simulink model "rpend_devdriv"  (R2018b)
settings: Solver=FixedStepDiscrete  StartTime=0.0  StopTime=999  FixedStep=0.01  RelTol=1e-3  EnableMultiTasking=on
values from neighbouring files (symbols this model uses):
  J = 0.000115    [init2.m]    (also in run_simulink_model.m)
  K = lqr(A, B, Q, R)    [run_simulink_model.m]
  mgl = 4    [init2.m]    (also in run_simulink_model.m)
  SP = [0,0,0,0]    [init2.m]    (also in run_simulink_model.m = [0, 0, 0, 0])
settings Model: SimulationMode=external  ExtModeTrigDuration=30000  Creator=user  LastModifiedBy=Student
settings DataIOCC: SaveFormat=Array  SignalLoggingSaveFormat=ModelDataLogs
settings OptimizationCC: ExpressionDepthLimit=2147483647  LifeSpan=inf
settings DebuggingCC: UnderspecifiedInitializationDetection=Classic  MergeDetectMultiDrivingBlocksExec=none  SolverPrmCheckMsg=warning  FcnCallInpInsideContextMsg=warning  StateNameClashWarn=warning  SFUnexpectedBacktrackingDiag=warning  SFNoUnconditionalDefaultTransitionDiag=warning  SFExecutionAtInitializationDiag=none
settings HardwareCC: ProdBitPerPointer=32  ProdBitPerSizeT=32  ProdBitPerPtrDiffT=32  ProdLargestAtomicFloat=None  ProdIntDivRoundTo=Undefined  ProdEndianess=Unspecified  ProdWordSize=32  ProdHWDeviceType=32-bit Generic
settings ModelReferenceCC: PropagateSignalLabelsOutOfModel=off
settings SFSimCC: SimUseLocalCustomCode=off
settings RTWCC: SystemTargetFile=rtcon_rpend_usb2.tlc  TemplateMakefile=rtcon_rpend_vc_usb2_x64.tmf  Description=rpend RTDAC/USB2 (Visual C/C++)  RTWUseLocalCustomCode=off
settings CodeAppCC: StateflowObjectComments=on
settings STFCustomTargetCC: ModelReferenceCompliant=off  GeneratePreprocessorConditionals=Disable all  CombineOutputUpdateFcns=on  MatFileLogging=on  SystemTargetFile=rtcon_rpend_usb2.tlc
settings GRTTargetCC: TargetLangStandard=C89/C90 (ANSI)  ModelReferenceCompliant=off  ParMdlRefBuildCompliant=off  CompOptLevelCompliant=off  ConcurrentExecutionCompliant=off  GeneratePreprocessorConditionals=Disable all  CPPClassGenCompliant=off  UseToolchainInfoCompliant=off  ExtMode=on  ExtModeMexFile=rtcon_ext_comm
settings ConfigComp: CovMetricSettings=dw  CovHtmlReporting=on  CovSaveCumulativeToWorkspaceVar=on  CovSaveSingleToWorkspaceVar=on  CovExternalEMLEnable=off  CovSFcnEnable=off

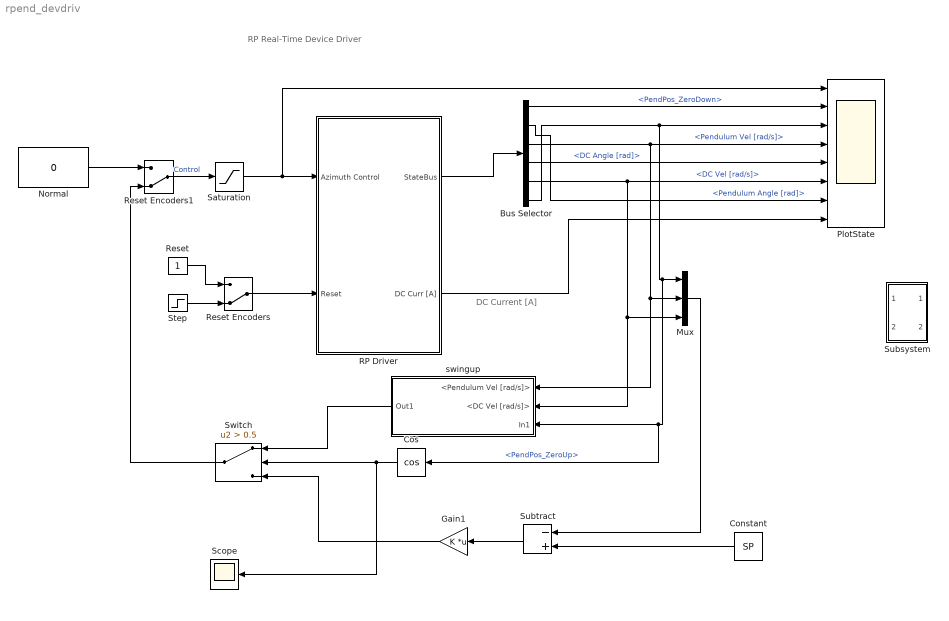
== system rpend_devdriv ==
  note: DC Current [A]
  note: RP Real-Time Device Driver
  Bus Selector : BusSelector  OutputSignals=PendPos_ZeroDown,Pendulum Angle [rad],Pendulum Vel [rad/s],DC Angle [rad],DC Vel [rad/s],PendPos_ZeroUp
  Constant : Constant  Value=SP
  Cos : Trigonometry  Operator=cos
  Gain1 : Gain  Gain=K  Multiplication=Matrix(K*u)
  Mux : Mux  Inputs=3
  Normal : Constant  Value=0
  PlotState : Scope  NumInputPorts=8
  RP Driver : Subsystem
      mask Display: image(imread('rwp.JPG'))
  Reset : Constant
  Reset Encoders : ManualSwitch  CurrentSetting=0
  Reset Encoders1 : ManualSwitch  CurrentSetting=0
  Saturation : Saturate  UpperLimit=0.9  LowerLimit=-0.9
  Scope : Scope
  Step : Step  Time=0.05  Before=1  After=0  SampleTime=0.01
  Subsystem : Subsystem
  Subtract : Sum  Inputs=-+
  Switch : Switch  Criteria=u2 > Threshold  Threshold=0.5
  swingup : Subsystem
  wires:
  Reset/1 -> Reset Encoders/1
  Reset Encoders/1 -> RP Driver/2(Reset)
  RP Driver/1(StateBus) -> Bus Selector/1
  Reset Encoders1/1 -> Saturation/1  "Control"
  Step/1 -> Reset Encoders/2
  Bus Selector/2 -> PlotState/7  "<Pendulum Angle [rad]>"
  Bus Selector/6 -> Cos/1, swingup/3(In1), Mux/1, PlotState/3  "<PendPos_ZeroUp>"
  Bus Selector/1 -> PlotState/2  "<PendPos_ZeroDown>"
  Bus Selector/5 -> Mux/3, swingup/2(<DC Vel [rad/s]>), PlotState/6  "<DC Vel [rad/s]>"
  Bus Selector/3 -> Mux/2, swingup/1(<Pendulum Vel [rad/s]>), PlotState/4  "<Pendulum Vel [rad/s]>"
  Bus Selector/4 -> PlotState/5  "<DC Angle [rad]>"
  RP Driver/2(DC Curr [A]) -> PlotState/8
  Mux/1 -> Subtract/1
  Constant/1 -> Subtract/2
  Saturation/1 -> RP Driver/1(Azimuth Control), PlotState/1
  Subtract/1 -> Gain1/1
  Normal/1 -> Reset Encoders1/1
  Switch/1 -> Reset Encoders1/2
  Cos/1 -> Scope/1, Switch/2
  Gain1/1 -> Switch/3
  swingup/1(Out1) -> Switch/1

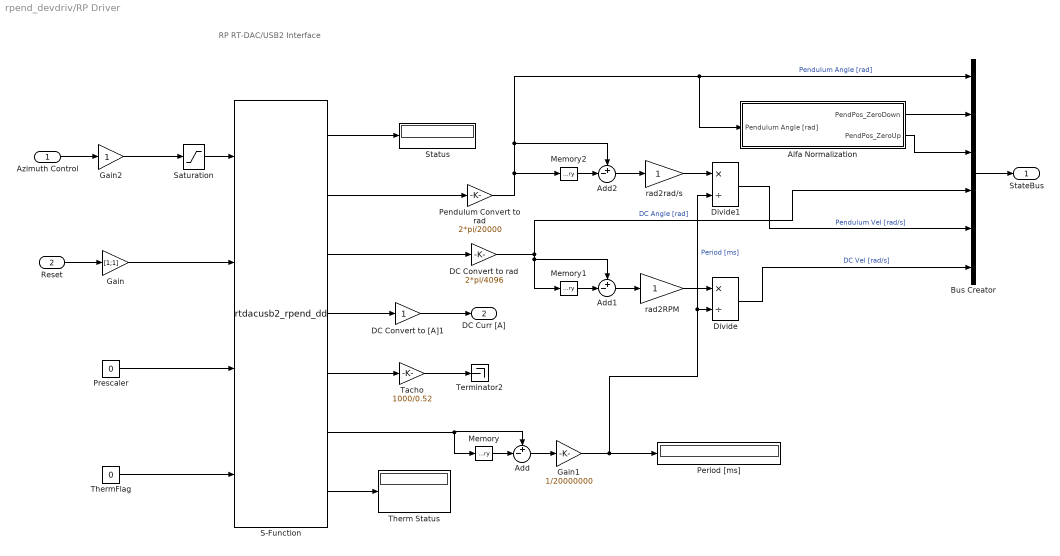
== system rpend_devdriv/RP Driver ==
  note: RP RT-DAC/USB2
      | Interface
  Azimuth Control : Inport
  Reset : Inport  Port=2
  Add : Sum  Inputs=+-|
  Add1 : Sum  Inputs=+-|
  Add2 : Sum  Inputs=+-|
  Alfa Normalization : Subsystem
  Bus Creator : BusCreator  Inputs=6
  DC Convert to [A]1 : Gain  SaturateOnIntegerOverflow=on  OutDataTypeStr=Inherit: Same as input  ParamDataTypeStr=Inherit: Same as input
  DC Convert to rad : Gain  Gain=2*pi/4096  SaturateOnIntegerOverflow=on  OutDataTypeStr=Inherit: Same as input  ParamDataTypeStr=Inherit: Same as input
  Divide : Product  Inputs=*/
  Divide1 : Product  Inputs=*/
  Gain : Gain  Gain=[1;1]
  Gain1 : Gain  Gain=1/20000000
  Gain2 : Gain
  Memory : Memory
  Memory1 : Memory
  Memory2 : Memory
  Pendulum Convert to rad : Gain  Gain=2*pi/20000  SaturateOnIntegerOverflow=on  OutDataTypeStr=Inherit: Same as input  ParamDataTypeStr=Inherit: Same as input
  Period [ms] : Display
  Prescaler : Constant  Value=0
  S-Function : S-Function  FunctionName=rtdacusb2_rpend_dd  Parameters=1, 0.01  SFunctionDeploymentMode=off  EnableBusSupport=off
  Saturation : Saturate  UpperLimit=1  LowerLimit=-1
  Status : Display
  Tacho : Gain  Gain=1000/0.52  SaturateOnIntegerOverflow=on  OutDataTypeStr=Inherit: Same as input  ParamDataTypeStr=Inherit: Same as input
  Terminator2 : Terminator
  Therm Status : Display
  ThermFlag : Constant  Value=0
  rad2RPM : Gain  SaturateOnIntegerOverflow=on  OutDataTypeStr=Inherit: Same as input  ParamDataTypeStr=Inherit: Same as input
  rad2rad/s : Gain  SaturateOnIntegerOverflow=on  OutDataTypeStr=Inherit: Same as input  ParamDataTypeStr=Inherit: Same as input
  StateBus : Outport
  DC Curr [A] : Outport  Port=2
  wires:
  Azimuth Control/1 -> Gain2/1
  Reset/1 -> Gain/1
  Saturation/1 -> S-Function/1
  S-Function/1 -> Status/1
  Pendulum Convert to rad/1 -> Memory2/1, Add2/1, Alfa Normalization/1(Pendulum Angle [rad]), Bus Creator/1  "Pendulum Angle [rad]"
  DC Convert to rad/1 -> Bus Creator/4, Add1/1, Memory1/1  "DC Angle [rad]"
  Memory/1 -> Add/2
  Add/1 -> Gain1/1
  Gain1/1 -> Divide1/2, Divide/2, Period [ms]/1  "Period [ms]"
  Gain2/1 -> Saturation/1
  S-Function/6 -> Memory/1, Add/1
  Tacho/1 -> Terminator2/1
  Memory1/1 -> Add1/2
  Add1/1 -> rad2RPM/1
  rad2RPM/1 -> Divide/1
  Memory2/1 -> Add2/2
  Add2/1 -> rad2rad/s/1
  rad2rad/s/1 -> Divide1/1
  Bus Creator/1 -> StateBus/1
  Alfa Normalization/1(PendPos_ZeroDown) -> Bus Creator/2
  Alfa Normalization/2(PendPos_ZeroUp) -> Bus Creator/3
  Divide1/1 -> Bus Creator/5  "Pendulum Vel [rad/s]"
  Divide/1 -> Bus Creator/6  "DC Vel [rad/s]"
  DC Convert to [A]1/1 -> DC Curr [A]/1
  Gain/1 -> S-Function/2
  Prescaler/1 -> S-Function/3
  ThermFlag/1 -> S-Function/4
  S-Function/4 -> DC Convert to [A]1/1
  S-Function/5 -> Tacho/1
  S-Function/7 -> Therm Status/1
  S-Function/2 -> Pendulum Convert to rad/1
  S-Function/3 -> DC Convert to rad/1

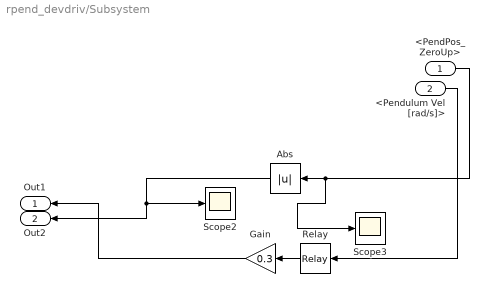
== system rpend_devdriv/Subsystem ==
  <PendPos_ZeroUp> : Inport
  <Pendulum Vel [rad/s]> : Inport  Port=2
  Abs : Abs
  Gain : Gain  Gain=0.3
  Relay : Relay  OnSwitchValue=0  OffSwitchValue=0  OnOutputValue=-1  OffOutputValue=1
  Scope2 : Scope
  Scope3 : Scope
  Out1 : Outport
  Out2 : Outport  Port=2
  wires:
  Gain/1 -> Out1/1
  <PendPos_ZeroUp>/1 -> Scope3/1, Abs/1
  Relay/1 -> Gain/1
  <Pendulum Vel [rad/s]>/1 -> Relay/1
  Abs/1 -> Out2/1, Scope2/1

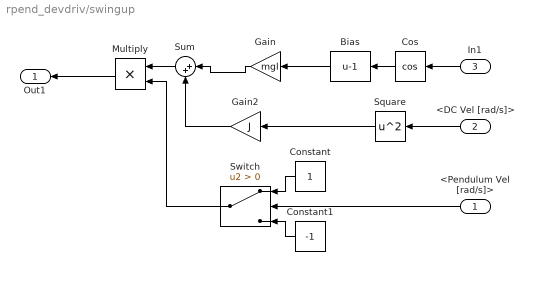
== system rpend_devdriv/swingup ==
  <Pendulum Vel [rad/s]> : Inport
  <DC Vel [rad/s]> : Inport  Port=2
  In1 : Inport  Port=3
  Bias : Bias  Bias=-1
  Constant : Constant
  Constant1 : Constant  Value=-1
  Cos : Trigonometry  Operator=cos
  Gain : Gain  Gain=mgl
  Gain2 : Gain  Gain=J
  Multiply : Product
  Square : Math  Operator=square  SaturateOnIntegerOverflow=on
  Sum : Sum  Inputs=|++
  Switch : Switch  Criteria=u2 > Threshold
  Out1 : Outport
  wires:
  Cos/1 -> Bias/1
  Bias/1 -> Gain/1
  <Pendulum Vel [rad/s]>/1 -> Switch/2
  Sum/1 -> Multiply/1
  Square/1 -> Gain2/1
  Gain/1 -> Sum/1
  Gain2/1 -> Sum/2
  <DC Vel [rad/s]>/1 -> Square/1
  Multiply/1 -> Out1/1
  Constant1/1 -> Switch/3
  Constant/1 -> Switch/1
  Switch/1 -> Multiply/2
  In1/1 -> Cos/1

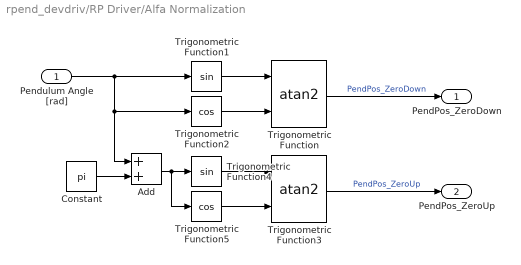
== system rpend_devdriv/RP Driver/Alfa Normalization ==
  Pendulum Angle [rad] : Inport
  Add : Sum
  Constant : Constant  Value=pi
  Trigonometric Function : Trigonometry  Operator=atan2
  Trigonometric Function1 : Trigonometry
  Trigonometric Function2 : Trigonometry  Operator=cos
  Trigonometric Function3 : Trigonometry  Operator=atan2
  Trigonometric Function4 : Trigonometry
  Trigonometric Function5 : Trigonometry  Operator=cos
  PendPos_ZeroDown : Outport
  PendPos_ZeroUp : Outport  Port=2
  wires:
  Trigonometric Function/1 -> PendPos_ZeroDown/1  "PendPos_ZeroDown"
  Pendulum Angle [rad]/1 -> Trigonometric Function1/1, Trigonometric Function2/1, Add/1
  Trigonometric Function1/1 -> Trigonometric Function/1
  Trigonometric Function2/1 -> Trigonometric Function/2
  Trigonometric Function3/1 -> PendPos_ZeroUp/1  "PendPos_ZeroUp"
  Trigonometric Function4/1 -> Trigonometric Function3/1
  Trigonometric Function5/1 -> Trigonometric Function3/2
  Add/1 -> Trigonometric Function5/1, Trigonometric Function4/1
  Constant/1 -> Add/2
